simulink model "controller_TRIAD_minimal"  (R2016b)
settings: Solver=VariableStepAuto  StartTime=0.0  StopTime=100  RelTol=1e-3
values from neighbouring files (symbols this model uses):
  quat_cmd = quat_cmd/norm(quat_cmd)    [ctrl_TRIAD_test.m]    (also in init_ctrl_TRIAD_test.m)
undefined symbols (not defined in the file or in its folder): sim_params
libraries: dynamics_lib x2, pd_control_lib x1, RW_assembly_simple_lib x1, command_processing x1, triad_coarse_estimator x1
settings Model: Creator=sexymathemagician  LastModifiedBy=sexymathemagician

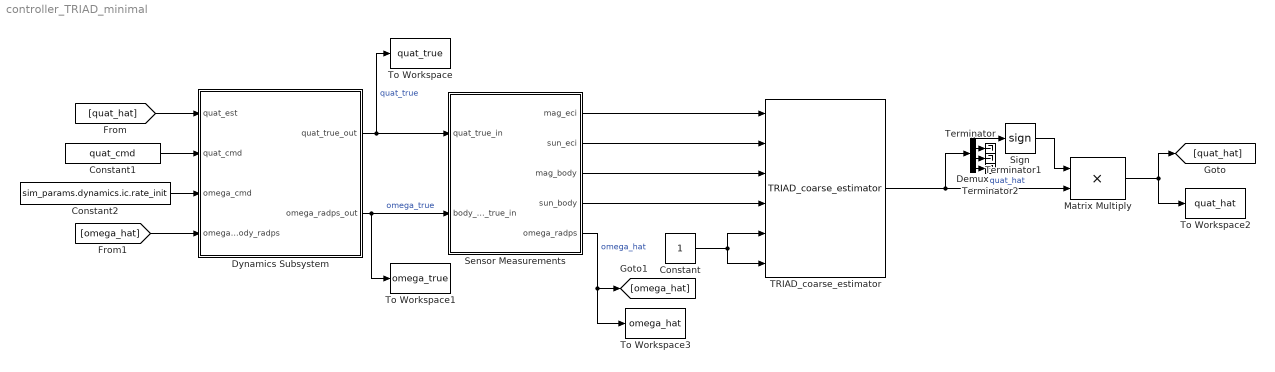
== system controller_TRIAD_minimal ==
  Constant : Constant
  Constant1 : Constant  Value=quat_cmd
  Constant2 : Constant  Value=sim_params.dynamics.ic.rate_init
  Demux : Demux
  Dynamics Subsystem : Subsystem
  Matrix Multiply : Product
  "Sensor Measurements " : Subsystem
  Sign : Signum
  TRIAD_coarse_estimator : triad_coarse_estimator/TRIAD_coarse_estimator
  Terminator : Terminator
  Terminator1 : Terminator
  Terminator2 : Terminator
  To Workspace : ToWorkspace  VariableName=quat_true  SaveFormat=Timeseries  SampleTime=-1
  To Workspace1 : ToWorkspace  VariableName=omega_true  SaveFormat=Timeseries  SampleTime=-1
  To Workspace2 : ToWorkspace  VariableName=quat_hat  SaveFormat=Timeseries  SampleTime=-1
  To Workspace3 : ToWorkspace  VariableName=omega_hat  SaveFormat=Timeseries  SampleTime=-1
  wires:
  "Sensor Measurements "/1(mag_eci) -> TRIAD_coarse_estimator/1
  "Sensor Measurements "/2(sun_eci) -> TRIAD_coarse_estimator/2
  "Sensor Measurements "/3(mag_body) -> TRIAD_coarse_estimator/3
  "Sensor Measurements "/4(sun_body) -> TRIAD_coarse_estimator/4
  Dynamics Subsystem/1(quat_true_out) -> To Workspace/1, "Sensor Measurements "/1(quat_true_in)  "quat_true"
  Dynamics Subsystem/2(omega_radps_out) -> To Workspace1/1, "Sensor Measurements "/2(body_rates_true_in)  "omega_true"
  [quat_hat] -> Dynamics Subsystem/1(quat_est)
  "Sensor Measurements "/5(omega_radps) -> To Workspace3/1, [omega_hat]  "omega_hat"
  [omega_hat] -> Dynamics Subsystem/4(omega_body_radps)
  Constant1/1 -> Dynamics Subsystem/2(quat_cmd)
  Constant2/1 -> Dynamics Subsystem/3("omega_cmd ")
  Constant/1 -> TRIAD_coarse_estimator/6, TRIAD_coarse_estimator/5
  TRIAD_coarse_estimator/1 -> Demux/1, Matrix Multiply/2  "quat_hat"
  Demux/2 -> Terminator/1
  Demux/3 -> Terminator1/1
  Demux/4 -> Terminator2/1
  Demux/1 -> Sign/1
  Sign/1 -> Matrix Multiply/1
  Matrix Multiply/1 -> To Workspace2/1, [quat_hat]

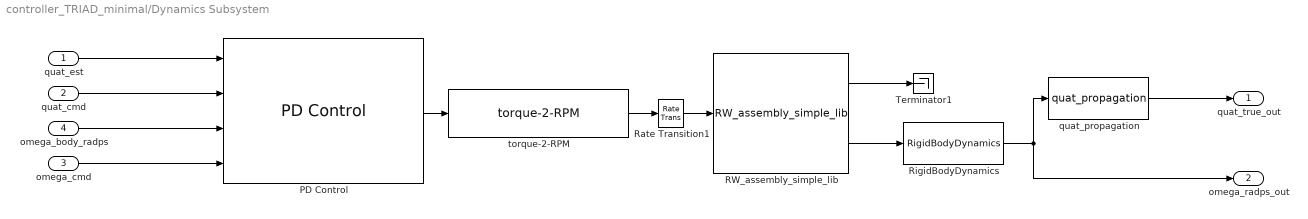
== system controller_TRIAD_minimal/Dynamics Subsystem ==
  quat_est : Inport
  quat_cmd : Inport  Port=2
  "omega_cmd " : Inport  Port=3
  omega_body_radps : Inport  Port=4
  PD Control : pd_control_lib/PD Control
  RW_assembly_simple_lib : RW_assembly_simple_lib/RW_assembly_simple_lib  natural_frequency=sim_params.actuators.reaction_wheel.natural_freq  damping_ratio=sim_params.actuators.reaction_wheel.damping  max_rate=sim_params.actuators.reaction_wheel.rate_limit
  Rate Transition1 : RateTransition  OutPortSampleTime=1/20
  RigidBodyDynamics : dynamics_lib/Dynamics/RigidBodyDynamics
  Terminator1 : Terminator
  quat_propagation : dynamics_lib/Dynamics/quat_propagation
  torque-2-RPM : command_processing/command_processing/torque-2-RPM
  quat_true_out : Outport
  omega_radps_out : Outport  Port=2
  wires:
  "omega_cmd "/1 -> PD Control/4
  quat_est/1 -> PD Control/1
  quat_cmd/1 -> PD Control/2
  omega_body_radps/1 -> PD Control/3
  torque-2-RPM/1 -> Rate Transition1/1
  Rate Transition1/1 -> RW_assembly_simple_lib/1
  RW_assembly_simple_lib/1 -> Terminator1/1
  RigidBodyDynamics/1 -> omega_radps_out/1, quat_propagation/1
  RW_assembly_simple_lib/2 -> RigidBodyDynamics/1
  quat_propagation/1 -> quat_true_out/1
  PD Control/1 -> torque-2-RPM/1

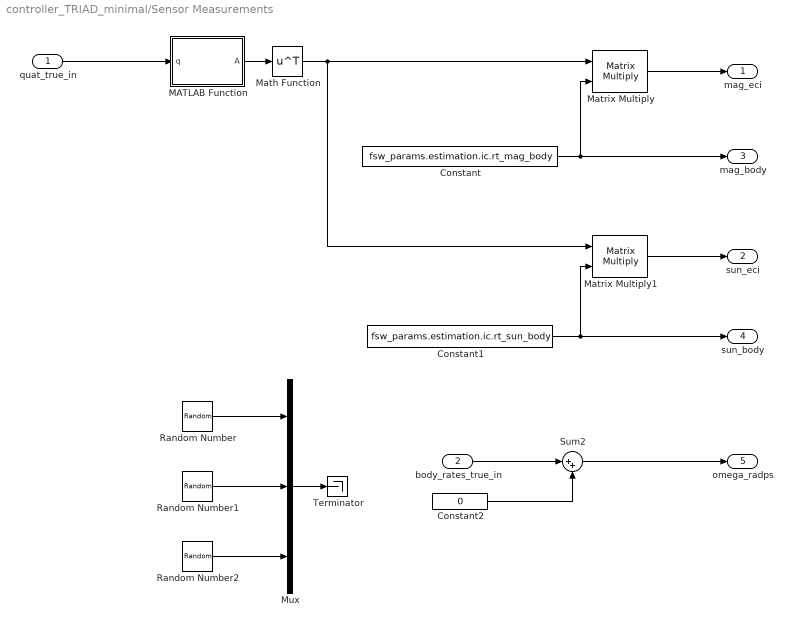
== system controller_TRIAD_minimal/Sensor Measurements  ==
  quat_true_in : Inport
  body_rates_true_in : Inport  Port=2
  Constant : Constant  Value=fsw_params.estimation.ic.rt_mag_body
  Constant1 : Constant  Value=fsw_params.estimation.ic.rt_sun_body
  Constant2 : Constant  Value=0
  MATLAB Function : MATLAB Function  TreatAsAtomicUnit=on
  Math Function : Math  Operator=transpose  SaturateOnIntegerOverflow=on
  Matrix Multiply : Product  Multiplication=Matrix(*)
  Matrix Multiply1 : Product  Multiplication=Matrix(*)
  Mux : Mux  Inputs=3
  Random Number : RandomNumber  Variance=(sim_params.sensors.gyro.arw)^2/(60*60)  SampleTime=0.1
  Random Number1 : RandomNumber  Variance=(sim_params.sensors.gyro.arw)^2/(60*60)  SampleTime=0.1
  Random Number2 : RandomNumber  Variance=(sim_params.sensors.gyro.arw)^2/(60*60)  SampleTime=0.1
  Sum2 : Sum  Inputs=|++
  Terminator : Terminator
  mag_eci : Outport
  sun_eci : Outport  Port=2
  mag_body : Outport  Port=3
  sun_body : Outport  Port=4
  omega_radps : Outport  Port=5
  wires:
  quat_true_in/1 -> MATLAB Function/1(q)
  Constant/1 -> Matrix Multiply/2, mag_body/1
  Matrix Multiply/1 -> mag_eci/1
  Constant1/1 -> Matrix Multiply1/2, sun_body/1
  Matrix Multiply1/1 -> sun_eci/1
  Random Number/1 -> Mux/1
  Random Number1/1 -> Mux/2
  Random Number2/1 -> Mux/3
  body_rates_true_in/1 -> Sum2/1
  Sum2/1 -> omega_radps/1
  Mux/1 -> Terminator/1
  Constant2/1 -> Sum2/2
  MATLAB Function/1(A) -> Math Function/1
  Math Function/1 -> Matrix Multiply1/1, Matrix Multiply/1

== matlab function controller_TRIAD_minimal/Sensor Measurements /MATLAB Function ==
  data: q input; A output
function A = quatToMatrix(q)
%#codegen

eta = q(1);
eps = q(2:4);

A = (2*eta^2 -1)*eye(3) + 2*(eps*eps') - 2*eta*skew(eps);


end

function cross = skew(a)
%#codegen

cross = [0 -a(3) a(2);
         a(3) 0 -a(1);
        -a(2) a(1) 0];

end
